simulink model "subjectVehicle"  (R2015b)
settings: Solver=ode3  SolverMode=SingleTasking  StartTime=0.0  StopTime=10.0  FixedStep=0.005  RelTol=1e-3
settings Model: Creator=Josef  LastModifiedBy=Josef
settings DataIOCC: SaveFormat=Array
settings OptimizationCC: BlockReduction=off  BooleanDataType=off
settings DebuggingCC: SaveWithParameterizedLinksMsg=none  SignalResolutionControl=TryResolveAllWithWarning
settings HardwareCC: ProdBitPerPointer=32  ProdWordSize=32  ProdHWDeviceType=Intel->x86-32 (Windows32)  TargetUnknown=on
settings ModelReferenceCC: ModelReferenceMinAlgLoopOccurrences=on
settings GRTTargetCC: GeneratePreprocessorConditionals=Disable all
settings ConfigComp: CovModelRefEnable=Off  CovSFcnEnable=off

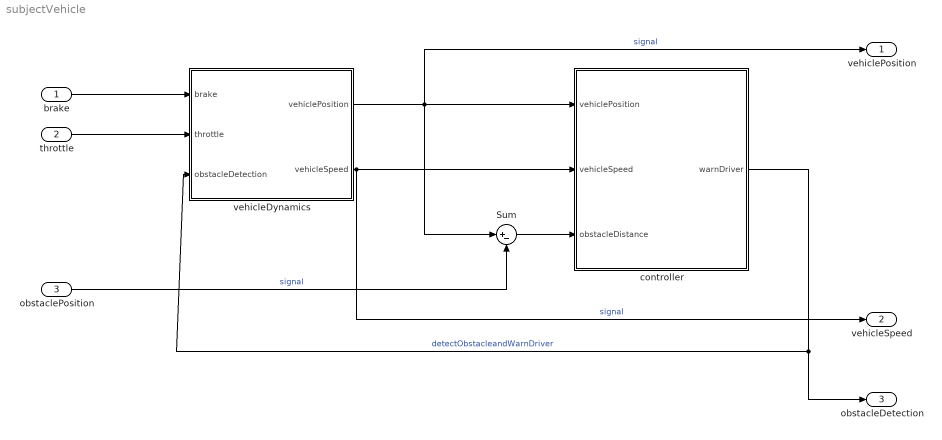
== system subjectVehicle ==
  brake : Inport
  throttle : Inport  Port=2
  obstaclePosition : Inport  Port=3
      settings: AttributesFormatString=signal
  Sum : Sum  Inputs=|+-
  controller : Subsystem
      settings: AttributesFormatString=CWS
  vehicleDynamics : Subsystem
  vehiclePosition : Outport
      settings: AttributesFormatString=signal
  vehicleSpeed : Outport  Port=2
      settings: AttributesFormatString=signal
  obstacleDetection : Outport  Port=3
      settings: AttributesFormatString=signal
  wires:
  vehicleDynamics/1(vehiclePosition) -> vehiclePosition/1, controller/1(vehiclePosition), Sum/1  "signal"
  vehicleDynamics/2(vehicleSpeed) -> vehicleSpeed/1, controller/2(vehicleSpeed)  "signal"
  controller/1(warnDriver) -> obstacleDetection/1, vehicleDynamics/3(obstacleDetection)  "detectObstacleandWarnDriver"
  throttle/1 -> vehicleDynamics/2(throttle)
  brake/1 -> vehicleDynamics/1(brake)
  Sum/1 -> controller/3(obstacleDistance)
  obstaclePosition/1 -> Sum/2  "signal"

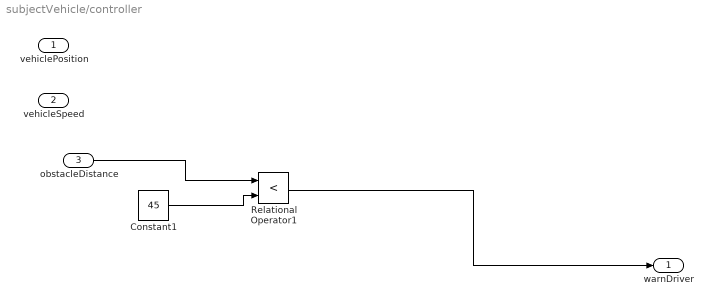
== system subjectVehicle/controller ==
  vehiclePosition : Inport
      settings: AttributesFormatString=signal
  vehicleSpeed : Inport  Port=2
      settings: AttributesFormatString=signal
  obstacleDistance : Inport  Port=3
      settings: AttributesFormatString=signal
  Constant1 : Constant  Value=45
  Relational Operator1 : RelationalOperator  Operator=<  OutDataTypeStr=boolean
  warnDriver : Outport
      settings: AttributesFormatString=detectObstacleandWarnDriver
  wires:
  obstacleDistance/1 -> Relational Operator1/1
  Constant1/1 -> Relational Operator1/2
  Relational Operator1/1 -> warnDriver/1

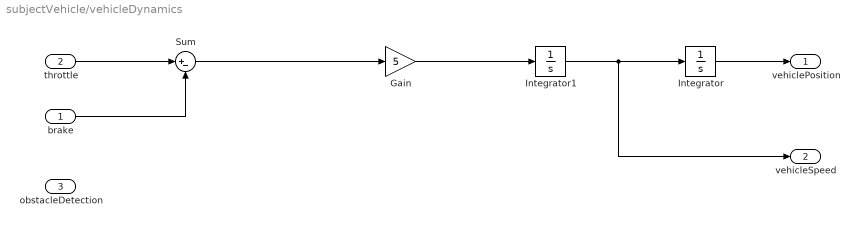
== system subjectVehicle/vehicleDynamics ==
  brake : Inport
  throttle : Inport  Port=2
  obstacleDetection : Inport  Port=3
      settings: AttributesFormatString=detectObstacleandWarnDriver
  Gain : Gain  Gain=5
  Integrator : Integrator
  Integrator1 : Integrator
  Sum : Sum  Inputs=|+-
  vehiclePosition : Outport
      settings: AttributesFormatString=signal
  vehicleSpeed : Outport  Port=2
      settings: AttributesFormatString=signal
  wires:
  Integrator/1 -> vehiclePosition/1
  Integrator1/1 -> vehicleSpeed/1, Integrator/1
  Gain/1 -> Integrator1/1
  Sum/1 -> Gain/1
  throttle/1 -> Sum/1
  brake/1 -> Sum/2
